simulink subsystem "control"  (R2025b)
settings: Solver=VariableStepAuto  StartTime=0.0  StopTime=10.0  RelTol=1e-3
libraries: slpidlib x4, simulink x2
settings Model: Creator=rowan  LastModifiedBy=rowan

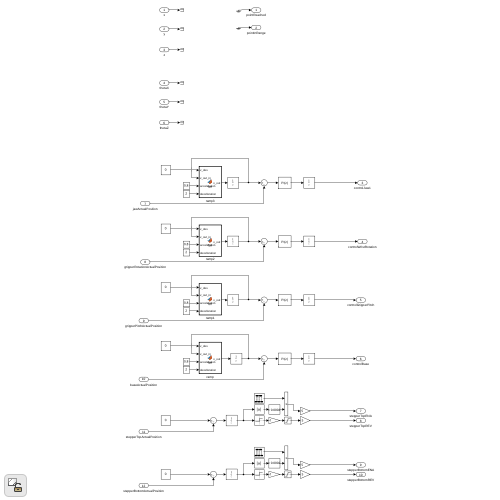
[thumbnail: Simulink's stored preview of the top-level diagram]
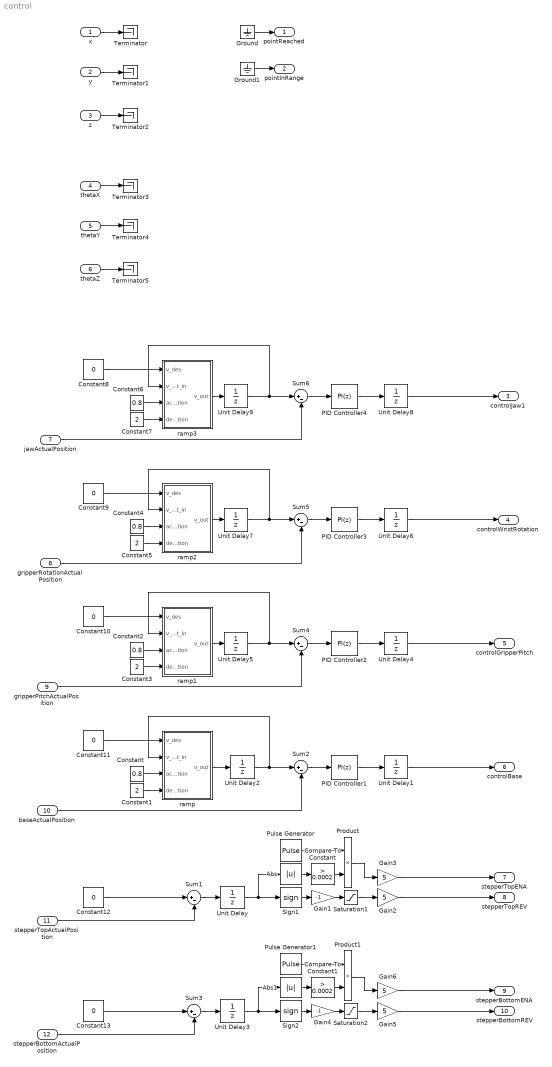
== system control ==
  x : Inport
  y : Inport  Port=2
  z : Inport  Port=3
  thetaX : Inport  Port=4
  thetaY : Inport  Port=5
  thetaZ : Inport  Port=6
  jawActualPosition : Inport  Port=7
  gripperRotationActualPosition : Inport  Port=8
  gripperPitchActualPosition : Inport  Port=9
  baseActualPosition : Inport  Port=10
  stepperTopActualPosition : Inport  Port=11
  stepperBottomActualPosition : Inport  Port=12
  Abs : Abs  SaturateOnIntegerOverflow=off
  Abs1 : Abs  SaturateOnIntegerOverflow=off
  Compare To Constant : simulink/Logic and Bit Operations/Compare To Constant  relop=>  const=0.0002  OutDataTypeStr=boolean
  Compare To Constant1 : simulink/Logic and Bit Operations/Compare To Constant  relop=>  const=0.0002  OutDataTypeStr=boolean
  Constant{,2,4,6} (4 alike) : Constant  Value=0.8
  Constant{1,3,5,7} (4 alike) : Constant  Value=2
  Constant{8..13} (6 alike) : Constant  Value=0
  Gain1 : Gain  Gain=-1
  Gain{2..3,5..6} (4 alike) : Gain  Gain=5
  Gain4 : Gain  Gain=-1
  Ground : Ground
  Ground1 : Ground
  PID Controller1 : slpidlib/PID Controller  Controller=PI  Form=Parallel  TimeDomain=Discrete-time  UseExternalTs=off  SampleTime=-1  IntegratorMethod=Forward Euler  FilterMethod=Forward Euler  ControllerParametersSource=internal  P=5  I=0.03  UseKiTs=off  D=1  UseExternalDerivativeSource=off  N=100  UseFilter=on  TunerSelectOption=Frequency Response Based  InitialConditionSource=internal  InitialConditionForIntegrator=0  InitialConditionForFilter=0  DifferentiatorICPrevScaledInput=0  ExternalReset=none  TrackingMode=off  Kt=1  LimitOutput=off  SatLimitsSource=internal  UpperSaturationLimit=inf  LowerSaturationLimit=-inf  LinearizeAsGain=on  AntiWindupMode=none  Kb=1  LimitIntegrator=off  UpperIntegratorSaturationLimit=inf  LowerIntegratorSaturationLimit=-inf  POutMin=[]  POutMax=[]  IOutMin=[]  IOutMax=[]  DOutMin=[]  DOutMax=[]  NOutMin=[]  NOutMax=[]  SumOutMin=[]  SumOutMax=[]  SaturationOutMin=[]  SaturationOutMax=[]  PParamMin=[]  PParamMax=[]  IParamMin=[]  IParamMax=[]  DParamMin=[]  DParamMax=[]  NParamMin=[]  NParamMax=[]  KbParamMin=[]  KbParamMax=[]  KtParamMin=[]  KtParamMax=[]  KbOutMin=[]  KbOutMax=[]  KtOutMin=[]  KtOutMax=[]  IntegratorOutMin=[]  IntegratorOutMax=[]  FilterOutMin=[]  FilterOutMax=[]  SumI1OutMin=[]  SumI1OutMax=[]  SumI2OutMin=[]  SumI2OutMax=[]  SumI3OutMin=[]  SumI3OutMax=[]  SumI4OutMin=[]  SumI4OutMax=[]  SumDOutMin=[]  SumDOutMax=[]  DifferentiatorOutMin=[]  DifferentiatorOutMax=[]  FilterDiffOutCoefMin=[]  FilterDiffOutCoefMax=[]  ReciprocalOutMin=[]  ReciprocalOutMax=[]  SumDenOutMin=[]  SumDenOutMax=[]  SumNumOutMin=[]  SumNumOutMax=[]  DivideOutMin=[]  DivideOutMax=[]  UdiffTsProdOutMin=[]  UdiffTsProdOutMax=[]  NTsProdOutMin=[]  NTsProdOutMax=[]  UintegralTsProdOutMin=[]  UintegralTsProdOutMax=[]  UngainTsProdOutMin=[]  UngainTsProdOutMax=[]  ClampingZeroOutDataTypeStr=Inherit: Inherit via back propagation  ClampingZeroOutMin=[]  ClampingZeroOutMax=[]  FilterDenConstantOutDataTypeStr=Inherit: Inherit via back propagation  FilterDenConstantOutMin=[]  FilterDenConstantOutMax=[]  PCopyOutDataTypeStr=Inherit: Inherit via back propagation  PCopyOutMin=[]  PCopyOutMax=[]  NCopyOutDataTypeStr=Inherit: Inherit via back propagation  NCopyOutMin=[]  NCopyOutMax=[]  IntegratorContinuousStateAttributes=''  IntegratorStateMustResolveToSignalObject=off  IntegratorRTWStateStorageClass=Auto  FilterContinuousStateAttributes=''  FilterStateMustResolveToSignalObject=off  FilterRTWStateStorageClass=Auto  ParallelPVariant=InternalParameters  IdealPVariant=Disabled  IVariant=InternalParameters  DVariant=Disabled  IntegratorVariant=Discrete  SatVariant=Disabled  AWVariant=Passthrough  PCopyVariant=Disabled  TRVariant=Disabled  FdbkBlocksVariant=Forward  IdealPFdbkVariant=Disabled  SatFdbkVariant=Disabled  DerivativeFilterVariant=Disabled  NVariant=Disabled  NCopyVariant=Disabled_SignalSpec  FilterICVariant=Disabled  IntegratorICVariant=InternalICs  ExternalResetVariant=Disabled  TRSumVariant=Passthrough  SumFdbkVariant=Disabled  SumVariant=Sum_PI  TsampFilterVariant=InternalTs  TsampNgainVariant=Passthrough  TsampIntegralVariant=Disabled_SignalSpec  ExternalSaturationOutDataTypeStr=Inherit: Same as second input  DerivativeSourceVariant=Disabled  PreIntVariant=InternalPreInt
  PID Controller2 : slpidlib/PID Controller  Controller=PI  Form=Parallel  TimeDomain=Discrete-time  UseExternalTs=off  SampleTime=-1  IntegratorMethod=Forward Euler  FilterMethod=Forward Euler  ControllerParametersSource=internal  P=2  I=0.05  UseKiTs=off  D=1  UseExternalDerivativeSource=off  N=100  UseFilter=on  TunerSelectOption=Frequency Response Based  InitialConditionSource=internal  InitialConditionForIntegrator=0  InitialConditionForFilter=0  DifferentiatorICPrevScaledInput=0  ExternalReset=none  TrackingMode=off  Kt=1  LimitOutput=off  SatLimitsSource=internal  UpperSaturationLimit=inf  LowerSaturationLimit=-inf  LinearizeAsGain=on  AntiWindupMode=none  Kb=1  LimitIntegrator=off  UpperIntegratorSaturationLimit=inf  LowerIntegratorSaturationLimit=-inf  POutMin=[]  POutMax=[]  IOutMin=[]  IOutMax=[]  DOutMin=[]  DOutMax=[]  NOutMin=[]  NOutMax=[]  SumOutMin=[]  SumOutMax=[]  SaturationOutMin=[]  SaturationOutMax=[]  PParamMin=[]  PParamMax=[]  IParamMin=[]  IParamMax=[]  DParamMin=[]  DParamMax=[]  NParamMin=[]  NParamMax=[]  KbParamMin=[]  KbParamMax=[]  KtParamMin=[]  KtParamMax=[]  KbOutMin=[]  KbOutMax=[]  KtOutMin=[]  KtOutMax=[]  IntegratorOutMin=[]  IntegratorOutMax=[]  FilterOutMin=[]  FilterOutMax=[]  SumI1OutMin=[]  SumI1OutMax=[]  SumI2OutMin=[]  SumI2OutMax=[]  SumI3OutMin=[]  SumI3OutMax=[]  SumI4OutMin=[]  SumI4OutMax=[]  SumDOutMin=[]  SumDOutMax=[]  DifferentiatorOutMin=[]  DifferentiatorOutMax=[]  FilterDiffOutCoefMin=[]  FilterDiffOutCoefMax=[]  ReciprocalOutMin=[]  ReciprocalOutMax=[]  SumDenOutMin=[]  SumDenOutMax=[]  SumNumOutMin=[]  SumNumOutMax=[]  DivideOutMin=[]  DivideOutMax=[]  UdiffTsProdOutMin=[]  UdiffTsProdOutMax=[]  NTsProdOutMin=[]  NTsProdOutMax=[]  UintegralTsProdOutMin=[]  UintegralTsProdOutMax=[]  UngainTsProdOutMin=[]  UngainTsProdOutMax=[]  ClampingZeroOutDataTypeStr=Inherit: Inherit via back propagation  ClampingZeroOutMin=[]  ClampingZeroOutMax=[]  FilterDenConstantOutDataTypeStr=Inherit: Inherit via back propagation  FilterDenConstantOutMin=[]  FilterDenConstantOutMax=[]  PCopyOutDataTypeStr=Inherit: Inherit via back propagation  PCopyOutMin=[]  PCopyOutMax=[]  NCopyOutDataTypeStr=Inherit: Inherit via back propagation  NCopyOutMin=[]  NCopyOutMax=[]  IntegratorContinuousStateAttributes=''  IntegratorStateMustResolveToSignalObject=off  IntegratorRTWStateStorageClass=Auto  FilterContinuousStateAttributes=''  FilterStateMustResolveToSignalObject=off  FilterRTWStateStorageClass=Auto  ParallelPVariant=InternalParameters  IdealPVariant=Disabled  IVariant=InternalParameters  DVariant=Disabled  IntegratorVariant=Discrete  SatVariant=Disabled  AWVariant=Passthrough  PCopyVariant=Disabled  TRVariant=Disabled  FdbkBlocksVariant=Forward  IdealPFdbkVariant=Disabled  SatFdbkVariant=Disabled  DerivativeFilterVariant=Disabled  NVariant=Disabled  NCopyVariant=Disabled_SignalSpec  FilterICVariant=Disabled  IntegratorICVariant=InternalICs  ExternalResetVariant=Disabled  TRSumVariant=Passthrough  SumFdbkVariant=Disabled  SumVariant=Sum_PI  TsampFilterVariant=InternalTs  TsampNgainVariant=Passthrough  TsampIntegralVariant=Disabled_SignalSpec  ExternalSaturationOutDataTypeStr=Inherit: Same as second input  DerivativeSourceVariant=Disabled  PreIntVariant=InternalPreInt
  PID Controller3 : slpidlib/PID Controller  Controller=PI  Form=Parallel  TimeDomain=Discrete-time  UseExternalTs=off  SampleTime=-1  IntegratorMethod=Forward Euler  FilterMethod=Forward Euler  ControllerParametersSource=internal  P=5  I=0.125  UseKiTs=off  D=1  UseExternalDerivativeSource=off  N=100  UseFilter=on  TunerSelectOption=Frequency Response Based  InitialConditionSource=internal  InitialConditionForIntegrator=0  InitialConditionForFilter=0  DifferentiatorICPrevScaledInput=0  ExternalReset=none  TrackingMode=off  Kt=1  LimitOutput=off  SatLimitsSource=internal  UpperSaturationLimit=inf  LowerSaturationLimit=-inf  LinearizeAsGain=on  AntiWindupMode=none  Kb=1  LimitIntegrator=off  UpperIntegratorSaturationLimit=inf  LowerIntegratorSaturationLimit=-inf  POutMin=[]  POutMax=[]  IOutMin=[]  IOutMax=[]  DOutMin=[]  DOutMax=[]  NOutMin=[]  NOutMax=[]  SumOutMin=[]  SumOutMax=[]  SaturationOutMin=[]  SaturationOutMax=[]  PParamMin=[]  PParamMax=[]  IParamMin=[]  IParamMax=[]  DParamMin=[]  DParamMax=[]  NParamMin=[]  NParamMax=[]  KbParamMin=[]  KbParamMax=[]  KtParamMin=[]  KtParamMax=[]  KbOutMin=[]  KbOutMax=[]  KtOutMin=[]  KtOutMax=[]  IntegratorOutMin=[]  IntegratorOutMax=[]  FilterOutMin=[]  FilterOutMax=[]  SumI1OutMin=[]  SumI1OutMax=[]  SumI2OutMin=[]  SumI2OutMax=[]  SumI3OutMin=[]  SumI3OutMax=[]  SumI4OutMin=[]  SumI4OutMax=[]  SumDOutMin=[]  SumDOutMax=[]  DifferentiatorOutMin=[]  DifferentiatorOutMax=[]  FilterDiffOutCoefMin=[]  FilterDiffOutCoefMax=[]  ReciprocalOutMin=[]  ReciprocalOutMax=[]  SumDenOutMin=[]  SumDenOutMax=[]  SumNumOutMin=[]  SumNumOutMax=[]  DivideOutMin=[]  DivideOutMax=[]  UdiffTsProdOutMin=[]  UdiffTsProdOutMax=[]  NTsProdOutMin=[]  NTsProdOutMax=[]  UintegralTsProdOutMin=[]  UintegralTsProdOutMax=[]  UngainTsProdOutMin=[]  UngainTsProdOutMax=[]  ClampingZeroOutDataTypeStr=Inherit: Inherit via back propagation  ClampingZeroOutMin=[]  ClampingZeroOutMax=[]  FilterDenConstantOutDataTypeStr=Inherit: Inherit via back propagation  FilterDenConstantOutMin=[]  FilterDenConstantOutMax=[]  PCopyOutDataTypeStr=Inherit: Inherit via back propagation  PCopyOutMin=[]  PCopyOutMax=[]  NCopyOutDataTypeStr=Inherit: Inherit via back propagation  NCopyOutMin=[]  NCopyOutMax=[]  IntegratorContinuousStateAttributes=''  IntegratorStateMustResolveToSignalObject=off  IntegratorRTWStateStorageClass=Auto  FilterContinuousStateAttributes=''  FilterStateMustResolveToSignalObject=off  FilterRTWStateStorageClass=Auto  ParallelPVariant=InternalParameters  IdealPVariant=Disabled  IVariant=InternalParameters  DVariant=Disabled  IntegratorVariant=Discrete  SatVariant=Disabled  AWVariant=Passthrough  PCopyVariant=Disabled  TRVariant=Disabled  FdbkBlocksVariant=Forward  IdealPFdbkVariant=Disabled  SatFdbkVariant=Disabled  DerivativeFilterVariant=Disabled  NVariant=Disabled  NCopyVariant=Disabled_SignalSpec  FilterICVariant=Disabled  IntegratorICVariant=InternalICs  ExternalResetVariant=Disabled  TRSumVariant=Passthrough  SumFdbkVariant=Disabled  SumVariant=Sum_PI  TsampFilterVariant=InternalTs  TsampNgainVariant=Passthrough  TsampIntegralVariant=Disabled_SignalSpec  ExternalSaturationOutDataTypeStr=Inherit: Same as second input  DerivativeSourceVariant=Disabled  PreIntVariant=InternalPreInt
  PID Controller4 : slpidlib/PID Controller  Controller=PI  Form=Parallel  TimeDomain=Discrete-time  UseExternalTs=off  SampleTime=-1  IntegratorMethod=Forward Euler  FilterMethod=Forward Euler  ControllerParametersSource=internal  P=5  I=0.125  UseKiTs=off  D=1  UseExternalDerivativeSource=off  N=100  UseFilter=on  TunerSelectOption=Frequency Response Based  InitialConditionSource=internal  InitialConditionForIntegrator=0  InitialConditionForFilter=0  DifferentiatorICPrevScaledInput=0  ExternalReset=none  TrackingMode=off  Kt=1  LimitOutput=off  SatLimitsSource=internal  UpperSaturationLimit=inf  LowerSaturationLimit=-inf  LinearizeAsGain=on  AntiWindupMode=none  Kb=1  LimitIntegrator=off  UpperIntegratorSaturationLimit=inf  LowerIntegratorSaturationLimit=-inf  POutMin=[]  POutMax=[]  IOutMin=[]  IOutMax=[]  DOutMin=[]  DOutMax=[]  NOutMin=[]  NOutMax=[]  SumOutMin=[]  SumOutMax=[]  SaturationOutMin=[]  SaturationOutMax=[]  PParamMin=[]  PParamMax=[]  IParamMin=[]  IParamMax=[]  DParamMin=[]  DParamMax=[]  NParamMin=[]  NParamMax=[]  KbParamMin=[]  KbParamMax=[]  KtParamMin=[]  KtParamMax=[]  KbOutMin=[]  KbOutMax=[]  KtOutMin=[]  KtOutMax=[]  IntegratorOutMin=[]  IntegratorOutMax=[]  FilterOutMin=[]  FilterOutMax=[]  SumI1OutMin=[]  SumI1OutMax=[]  SumI2OutMin=[]  SumI2OutMax=[]  SumI3OutMin=[]  SumI3OutMax=[]  SumI4OutMin=[]  SumI4OutMax=[]  SumDOutMin=[]  SumDOutMax=[]  DifferentiatorOutMin=[]  DifferentiatorOutMax=[]  FilterDiffOutCoefMin=[]  FilterDiffOutCoefMax=[]  ReciprocalOutMin=[]  ReciprocalOutMax=[]  SumDenOutMin=[]  SumDenOutMax=[]  SumNumOutMin=[]  SumNumOutMax=[]  DivideOutMin=[]  DivideOutMax=[]  UdiffTsProdOutMin=[]  UdiffTsProdOutMax=[]  NTsProdOutMin=[]  NTsProdOutMax=[]  UintegralTsProdOutMin=[]  UintegralTsProdOutMax=[]  UngainTsProdOutMin=[]  UngainTsProdOutMax=[]  ClampingZeroOutDataTypeStr=Inherit: Inherit via back propagation  ClampingZeroOutMin=[]  ClampingZeroOutMax=[]  FilterDenConstantOutDataTypeStr=Inherit: Inherit via back propagation  FilterDenConstantOutMin=[]  FilterDenConstantOutMax=[]  PCopyOutDataTypeStr=Inherit: Inherit via back propagation  PCopyOutMin=[]  PCopyOutMax=[]  NCopyOutDataTypeStr=Inherit: Inherit via back propagation  NCopyOutMin=[]  NCopyOutMax=[]  IntegratorContinuousStateAttributes=''  IntegratorStateMustResolveToSignalObject=off  IntegratorRTWStateStorageClass=Auto  FilterContinuousStateAttributes=''  FilterStateMustResolveToSignalObject=off  FilterRTWStateStorageClass=Auto  ParallelPVariant=InternalParameters  IdealPVariant=Disabled  IVariant=InternalParameters  DVariant=Disabled  IntegratorVariant=Discrete  SatVariant=Disabled  AWVariant=Passthrough  PCopyVariant=Disabled  TRVariant=Disabled  FdbkBlocksVariant=Forward  IdealPFdbkVariant=Disabled  SatFdbkVariant=Disabled  DerivativeFilterVariant=Disabled  NVariant=Disabled  NCopyVariant=Disabled_SignalSpec  FilterICVariant=Disabled  IntegratorICVariant=InternalICs  ExternalResetVariant=Disabled  TRSumVariant=Passthrough  SumFdbkVariant=Disabled  SumVariant=Sum_PI  TsampFilterVariant=InternalTs  TsampNgainVariant=Passthrough  TsampIntegralVariant=Disabled_SignalSpec  ExternalSaturationOutDataTypeStr=Inherit: Same as second input  DerivativeSourceVariant=Disabled  PreIntVariant=InternalPreInt
  Product : Product
  Product1 : Product
  Pulse Generator : DiscretePulseGenerator  SampleTime=0.001
  Pulse Generator1 : DiscretePulseGenerator  SampleTime=0.001
  Saturation1 : Saturate  UpperLimit=1  LowerLimit=0
  Saturation2 : Saturate  UpperLimit=1  LowerLimit=0
  Sign1 : Signum
  Sign2 : Signum
  Sum{1..6} (6 alike) : Sum  Inputs=|+-
  Terminator{,1..5} (6 alike) : Terminator
  Unit Delay{,1..9} (10 alike) : UnitDelay  SampleTime=-1  HasFrameUpgradeWarning=on
  ramp : MATLAB Function  TreatAsAtomicUnit=on
  ramp1 : MATLAB Function  TreatAsAtomicUnit=on
  ramp2 : MATLAB Function  TreatAsAtomicUnit=on
  ramp3 : MATLAB Function  TreatAsAtomicUnit=on
  pointReached : Outport
  pointInRange : Outport  Port=2
  controlJaw1 : Outport  Port=3
  controlWristRotation : Outport  Port=4
  controlGripperPitch : Outport  Port=5
  controlBase : Outport  Port=6
  stepperTopENA : Outport  Port=7
  stepperTopREV : Outport  Port=8
  stepperBottomENA : Outport  Port=9
  stepperBottomREV : Outport  Port=10
  wires:
  Unit Delay4/1 -> controlGripperPitch/1
  Unit Delay3/1 -> Abs1/1, Sign2/1
  Pulse Generator1/1 -> Product1/1
  Abs1/1 -> Compare To Constant1/1
  ramp1/1(v_out) -> Unit Delay5/1
  Gain5/1 -> stepperBottomREV/1
  Product1/1 -> Gain6/1
  PID Controller2/1 -> Unit Delay4/1
  Constant/1 -> ramp/3(acceleration)
  Unit Delay2/1 -> ramp/2(v_out_in), Sum2/1
  Constant10/1 -> ramp1/1(v_des)
  Gain4/1 -> Saturation2/1
  ramp3/1(v_out) -> Unit Delay9/1
  Unit Delay8/1 -> controlJaw1/1
  Constant1/1 -> ramp/4(decelleration)
  Compare To Constant1/1 -> Product1/2
  Sum3/1 -> Unit Delay3/1
  PID Controller4/1 -> Unit Delay8/1
  Gain6/1 -> stepperBottomENA/1
  Constant7/1 -> ramp3/4(decelleration)
  PID Controller3/1 -> Unit Delay6/1
  Gain3/1 -> stepperTopENA/1
  Sum4/1 -> PID Controller2/1
  Constant9/1 -> ramp2/1(v_des)
  Unit Delay6/1 -> controlWristRotation/1
  ramp/1(v_out) -> Unit Delay2/1
  ramp2/1(v_out) -> Unit Delay7/1
  Unit Delay5/1 -> Sum4/1, ramp1/2(v_out_in)
  Unit Delay7/1 -> ramp2/2(v_out_in), Sum5/1
  Sign2/1 -> Gain4/1
  Gain2/1 -> stepperTopREV/1
  Constant4/1 -> ramp2/3(acceleration)
  Saturation2/1 -> Gain5/1
  Constant8/1 -> ramp3/1(v_des)
  Sum2/1 -> PID Controller1/1
  Constant5/1 -> ramp2/4(decelleration)
  Constant6/1 -> ramp3/3(acceleration)
  Constant13/1 -> Sum3/1
  Sum5/1 -> PID Controller3/1
  Unit Delay9/1 -> Sum6/1, ramp3/2(v_out_in)
  Sum6/1 -> PID Controller4/1
  Gain1/1 -> Saturation1/1
  Constant2/1 -> ramp1/3(acceleration)
  Constant3/1 -> ramp1/4(decelleration)
  Compare To Constant/1 -> Product/2
  Pulse Generator/1 -> Product/1
  Product/1 -> Gain3/1
  Sign1/1 -> Gain1/1
  Sum1/1 -> Unit Delay/1
  Abs/1 -> Compare To Constant/1
  Constant11/1 -> ramp/1(v_des)
  Unit Delay1/1 -> controlBase/1
  Saturation1/1 -> Gain2/1
  PID Controller1/1 -> Unit Delay1/1
  Constant12/1 -> Sum1/1
  Unit Delay/1 -> Sign1/1, Abs/1
  baseActualPosition/1 -> Sum2/2
  stepperBottomActualPosition/1 -> Sum3/2
  stepperTopActualPosition/1 -> Sum1/2
  gripperPitchActualPosition/1 -> Sum4/2
  gripperRotationActualPosition/1 -> Sum5/2
  jawActualPosition/1 -> Sum6/2
  Ground/1 -> pointReached/1
  Ground1/1 -> pointInRange/1
  x/1 -> Terminator/1
  y/1 -> Terminator1/1
  z/1 -> Terminator2/1
  thetaX/1 -> Terminator3/1
  thetaY/1 -> Terminator4/1
  thetaZ/1 -> Terminator5/1

== matlab function control/ramp1 ==
  data: v_des input; v_out output; v_out_in input; acceleration input; decelleration input
function v_out = fcn(v_des, v_out_in, acceleration, decelleration)
sample_time = 0.001;

persistent v;
if isempty(v)
    v = zeros;  % initialize persistent velocity
end

if abs(v - v_des) < sample_time *acceleration 
    v_out = v;
    return;
end

if v_out_in < v_des
    v = v + acceleration * sample_time;
    if v > v_des
        v = v_des;
    end
else
    v = v - decelleration * sample_time;
    if v < 0
        v = 0;
    end
end

v_out = v;

== matlab function control/ramp2 ==
  data: v_des input; v_out output; v_out_in input; acceleration input; decelleration input
function v_out = fcn(v_des, v_out_in, acceleration, decelleration)
sample_time = 0.001;

persistent v;
if isempty(v)
    v = zeros;  % initialize persistent velocity
end

if abs(v - v_des) < sample_time *acceleration 
    v_out = v;
    return;
end

if v_out_in < v_des
    v = v + acceleration * sample_time;
    if v > v_des
        v = v_des;
    end
else
    v = v - decelleration * sample_time;
    if v < 0
        v = 0;
    end
end

v_out = v;

== matlab function control/ramp3 ==
  data: v_des input; v_out output; v_out_in input; acceleration input; decelleration input
function v_out = fcn(v_des, v_out_in, acceleration, decelleration)
sample_time = 0.001;

persistent v;
if isempty(v)
    v = zeros;  % initialize persistent velocity
end

if abs(v - v_des) < sample_time *acceleration 
    v_out = v;
    return;
end

if v_out_in < v_des
    v = v + acceleration * sample_time;
    if v > v_des
        v = v_des;
    end
else
    v = v - decelleration * sample_time;
    if v < 0
        v = 0;
    end
end

v_out = v;

== matlab function control/ramp ==
  data: v_des input; v_out output; v_out_in input; acceleration input; decelleration input
function v_out = fcn(v_des, v_out_in, acceleration, decelleration)
sample_time = 0.001;

persistent v;
if isempty(v)
    v = zeros;  % initialize persistent velocity
end

if abs(v - v_des) < sample_time *acceleration 
    v_out = v;
    return;
end

if v_out_in < v_des
    v = v + acceleration * sample_time;
    if v > v_des
        v = v_des;
    end
else
    v = v - decelleration * sample_time;
    if v < 0
        v = 0;
    end
end

v_out = v;
